simulink model "ejemplo_4"  (R2020b)
settings: Solver=VariableStepAuto  StartTime=0.0  StopTime=2.5  RelTol=1e-3
settings Model: Creator=carma  LastModifiedBy=carma

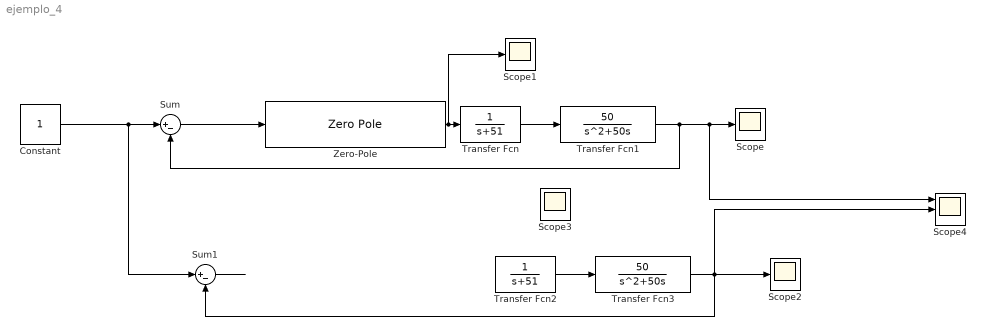
== system ejemplo_4 ==
  Constant : Constant  VectorParams1D=off  SampleTime=-1
  Scope{,1..3} (4 alike) : Scope
  Scope4 : Scope  NumInputPorts=3
  Sum : Sum  Inputs=|+-
  Sum1 : Sum  Inputs=|+-
  Transfer Fcn : TransferFcn  Denominator=[1 51]
  Transfer Fcn1 : TransferFcn  Numerator=[50]  Denominator=[1 50 0]
  Transfer Fcn2 : TransferFcn  Denominator=[1 51]
  Transfer Fcn3 : TransferFcn  Numerator=[50]  Denominator=[1 50 0]
  Zero-Pole : ZeroPole  Zeros=[-0.01 -8.18]  Poles=[-5 -0.0016]  Gain=250
  wires:
  Transfer Fcn/1 -> Transfer Fcn1/1
  Transfer Fcn1/1 -> Scope4/1, Scope/1, Sum/2
  Sum/1 -> Zero-Pole/1
  Zero-Pole/1 -> Scope1/1, Transfer Fcn/1
  Transfer Fcn3/1 -> Sum1/2, Scope4/2, Scope2/1
  Transfer Fcn2/1 -> Transfer Fcn3/1
  Constant/1 -> Sum1/1, Sum/1
  Sum1/1 -> ?
  ? -> Scope3/1, Transfer Fcn2/1
